simulink model "conversationhorn"  (R2018a)
settings: Solver=VariableStepAuto  StartTime=0.0  StopTime=10  RelTol=1e-3
libraries: dspvision x2, dspsnks4 x1, dspadpt3 x1
settings Model: Creator=Lenovo  LastModifiedBy=Lenovo

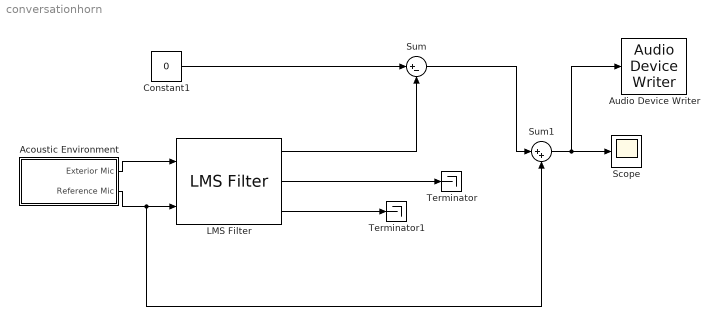
== system conversationhorn ==
  Acoustic Environment : Subsystem
  Audio Device Writer : dspsnks4/Audio Device Writer  Driver=DirectSound  Device=Default  InheritSampleRate=on  SampleRate=44100  BitDepth=16-bit integer  BufferSize=4096  NumBuffers=10  DefaultOutputChannelMapping=on  OutputChannelMapping=1:2  OutputNumUnderrunSamples=off  DriverIdx=1  DeviceWarnFlag=''
  Constant1 : Constant  Value=0
  LMS Filter : dspadpt3/LMS Filter  Algo=Normalized LMS  L=48  stepflag=Dialog  mu=0.005  leakage=1  ic=0  Adapt=off  resetflag=None  weights=on  secondCoeffMode=User-defined  secondCoeffWordLength=2  secondCoeffFracLength=15  accum2Mode=User-defined  accum2FracLength=20  prodOutput2Mode=User-defined  prodOutput2FracLength=20  prodOutput3Mode=User-defined  prodOutput3FracLength=20  prodOutput4Mode=User-defined  prodOutput4FracLength=20  quotientMode=User-defined  quotientFracLength=20  roundingMode=Floor  overflowMode=off  addnparflag=off
      settings: SourceProductName=DSP System Toolbox  SourceProductBaseCode=DS
  Scope : Scope
  Sum : Sum  Inputs=|+-
  Sum1 : Sum  Inputs=|++
  Terminator : Terminator
  Terminator1 : Terminator
  wires:
  LMS Filter/2 -> Terminator/1
  Acoustic Environment/1(Exterior Mic) -> LMS Filter/1
  Acoustic Environment/2(Reference Mic) -> LMS Filter/2, Sum1/2
  Constant1/1 -> Sum/1
  Sum/1 -> Sum1/1
  LMS Filter/3 -> Terminator1/1
  LMS Filter/1 -> Sum/2
  Sum1/1 -> Audio Device Writer/1, Scope/1

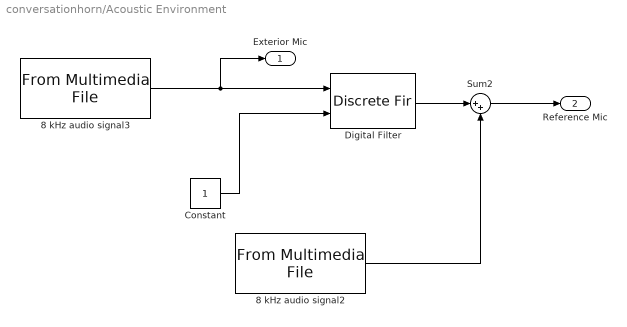
== system conversationhorn/Acoustic Environment ==
  8 kHz audio signal2 : dspvision/From Multimedia File  inputFilename=D:\downloads\mc12.wav  loop=on  numPlays=1  outputStreams=Audio only  videoDataType=single  audioDataType=single  inheritSampleTime=off  userDefinedSampleTime=1/500  noAudioOutput=off  isIntensityVideo=off  fourcc=RGB  colorVideoFormat=Separate color signals  outputEOF=off  dataOrg=Column-major  audioFrameSize=80  computeAudioFrameSize=off  outSamplingMode=Sample based
      settings: SourceProductBaseCode=VP
  8 kHz audio signal3 : dspvision/From Multimedia File  inputFilename=D:\downloads\mixkit-distant-train-horn-1654 (1).wav  loop=on  numPlays=1  outputStreams=Audio only  videoDataType=single  audioDataType=single  inheritSampleTime=off  userDefinedSampleTime=1/500  noAudioOutput=off  isIntensityVideo=off  fourcc=RGB  colorVideoFormat=Separate color signals  outputEOF=off  dataOrg=Column-major  audioFrameSize=80  computeAudioFrameSize=off  outSamplingMode=Sample based
      settings: SourceProductBaseCode=VP
  Constant : Constant  OutDataTypeStr=single
  Digital Filter : DiscreteFir  CoefSource=Input port  Coefficients=[1 2]  InputProcessing=Columns as channels (frame based)  AccumDataTypeStr=Inherit: Same as product output  OutDataTypeStr=Inherit: Same as input
      settings: InputPortMap=u0,u1
  Sum2 : Sum  Inputs=|++  SaturateOnIntegerOverflow=on  InputSameDT=on  OutDataTypeStr=Inherit: Same as first input
  Exterior Mic : Outport
  Reference Mic : Outport  Port=2
  wires:
  Digital Filter/1 -> Sum2/1
  Constant/1 -> Digital Filter/2
  8 kHz audio signal2/1 -> Sum2/2
  8 kHz audio signal3/1 -> Digital Filter/1, Exterior Mic/1
  Sum2/1 -> Reference Mic/1
